simulink subsystem "Integrator"  (R2023b)
settings: Solver=VariableStepAuto  StartTime=0.0  StopTime=10.0  RelTol=1e-3
undefined symbols (not defined in the file): DiscIntNeverNeededParam
settings Model: Creator=leona  LastModifiedBy=leona

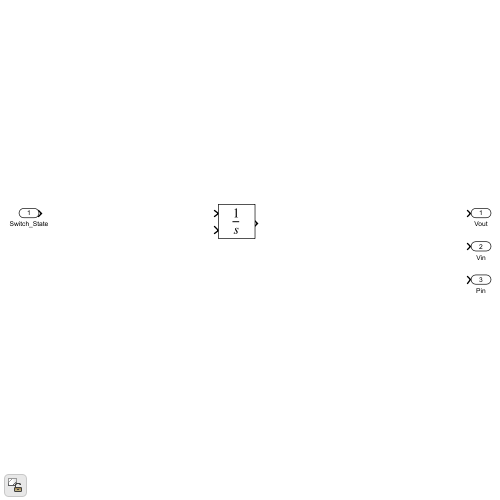
[thumbnail: Simulink's stored preview of the top-level diagram]
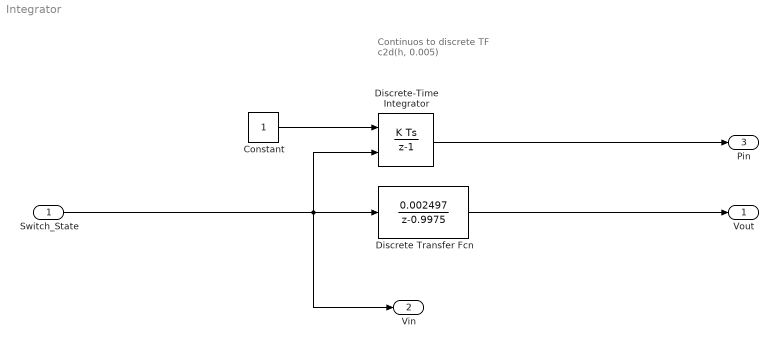
== system Integrator ==
  note: Continuos to discrete TF
      | c2d(h, 0.005)
  Switch_State : Inport
  Constant : Constant
  Discrete Transfer Fcn : DiscreteTransferFcn  Numerator=[0.002497]  Denominator=[1 -0.9975]
  Discrete-Time Integrator : DiscreteIntegrator  ExternalReset=level  SampleTime=-1  ICPrevOutput=DiscIntNeverNeededParam  ICPrevScaledInput=DiscIntNeverNeededParam
  Vout : Outport
  Vin : Outport  Port=2
  Pin : Outport  Port=3
  wires:
  Constant/1 -> Discrete-Time Integrator/1
  Switch_State/1 -> Discrete-Time Integrator/2, Discrete Transfer Fcn/1, Vin/1
  Discrete Transfer Fcn/1 -> Vout/1
  Discrete-Time Integrator/1 -> Pin/1
